simulink model "ex3_14"  (R2024a)
settings: Solver=ode4  StartTime=0.0  StopTime=tstop  FixedStep=tstop/1000  RelTol=1e-3
libraries: cstblocks x6
settings Model: Creator=mohammed  LastModifiedBy=mohammed
settings DataIOCC: ReturnWorkspaceOutputs=off

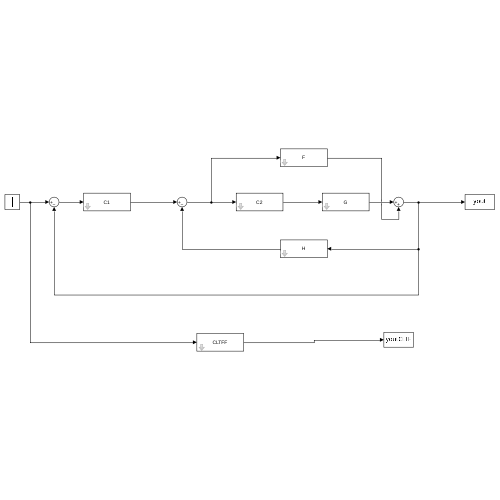
[thumbnail: Simulink's stored preview of the top-level diagram]
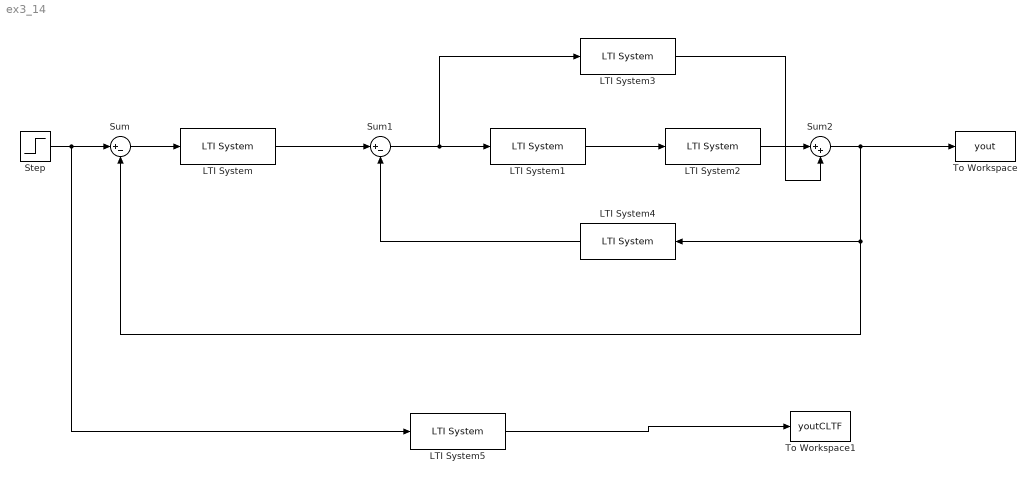
== system ex3_14 ==
  LTI System : cstblocks/LTI System  sys=C1  IC=[]  PadeOrder=0
  LTI System1 : cstblocks/LTI System  sys=C2  IC=[]  PadeOrder=0
  LTI System2 : cstblocks/LTI System  sys=G  IC=[]  PadeOrder=0
  LTI System3 : cstblocks/LTI System  sys=F  IC=[]  PadeOrder=0
  LTI System4 : cstblocks/LTI System  sys=H  IC=[]  PadeOrder=0
  LTI System5 : cstblocks/LTI System  sys=CLTFF  IC=[]  PadeOrder=0
  Step : Step  Time=0  SampleTime=0
  Sum : Sum  Inputs=|+-
  Sum1 : Sum  Inputs=|+-
  Sum2 : Sum  Inputs=|++
  To Workspace : ToWorkspace  VariableName=yout  SampleTime=-1
  To Workspace1 : ToWorkspace  VariableName=youtCLTF  SampleTime=-1
  wires:
  Step/1 -> LTI System5/1, Sum/1
  Sum/1 -> LTI System/1
  LTI System/1 -> Sum1/1
  Sum1/1 -> LTI System3/1, LTI System1/1
  LTI System4/1 -> Sum1/2
  LTI System1/1 -> LTI System2/1
  LTI System2/1 -> Sum2/1
  Sum2/1 -> LTI System4/1, Sum/2, To Workspace/1
  LTI System3/1 -> Sum2/2
  LTI System5/1 -> To Workspace1/1
